simulink model "mod3_thermalnoises"  (R2013a)
settings: Solver=FixedStepDiscrete  StartTime=0.0  StopTime=swpctrl.trantime  RelTol=1e-3
undefined symbols (not defined in the file): Fs, modctrl
libraries: dspsrcs4 x4, dspsigops x3
settings Model: Creator=amyles  LastModifiedBy=amyles
settings DataIOCC: LimitDataPoints=off  MaxDataPoints=50000  SignalLoggingSaveFormat=ModelDataLogs
settings OptimizationCC: InlineParams=on  ExpressionDepthLimit=2147483647
settings DebuggingCC: FcnCallInpInsideContextMsg=UseLocalSettings  StrictBusMsg=Warning
settings ModelReferenceCC: ModelReferenceNumInstancesAllowed=Single
settings GRTTargetCC: CombineOutputUpdateFcns=off  GRTInterface=on

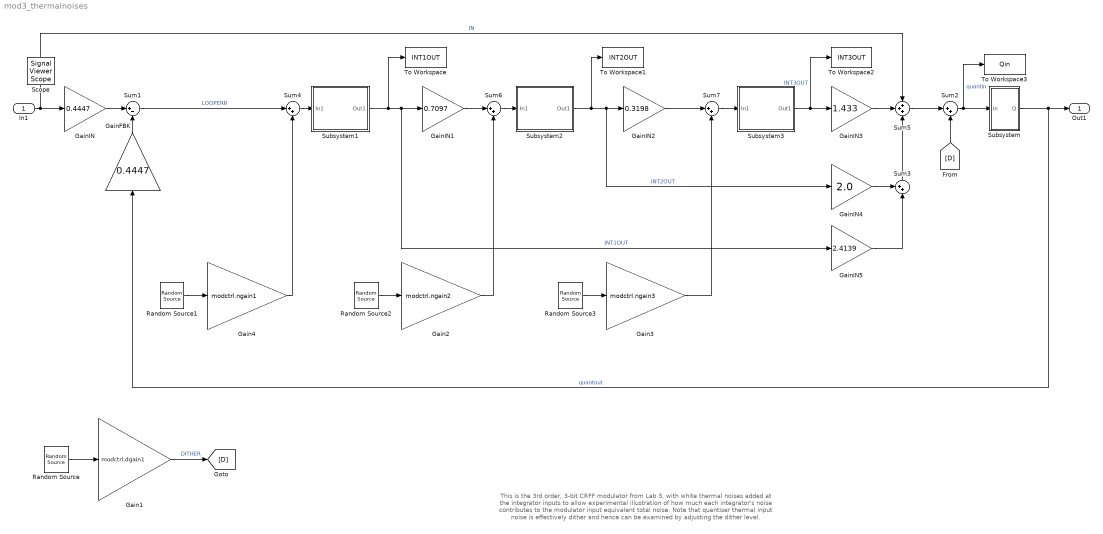
== system mod3_thermalnoises ==
  note: This is the 3rd order, 3-bit CRFF modulator from Lab 3, with
      | white thermal noises added at the integrator inputs to allow experimental
      | illustration of how much each integrator's noise contributes to the
      | modulator input equivalent total noise. Note that quantiser thermal input noise
      | is effectively dither and hence can be examined by adjusting the dither level.
  In1 : Inport
  Gain1 : Gain  Gain=modctrl.dgain1
      settings: AttributesFormatString=Dither level adjust
  Gain2 : Gain  Gain=modctrl.ngain2
  Gain3 : Gain  Gain=modctrl.ngain3
  Gain4 : Gain  Gain=modctrl.ngain1
  GainFBK : Gain  Gain=0.4447
  GainIN : Gain  Gain=0.4447
  GainIN1 : Gain  Gain=0.7097
  GainIN2 : Gain  Gain=0.3198
  GainIN3 : Gain  Gain=1.433
  GainIN4 : Gain  Gain=2.0
  GainIN5 : Gain  Gain=2.4139
  Random Source{,1..3} (4 alike) : dspsrcs4/Random Source  SrcType=Uniform  NormMethod=Ziggurat  CltLength=12  MinVal=-1  MaxVal=1  MeanVal=0  VarVal=1  RepMode=Not repeatable  rawSeed=1  IsInherit=off  SampMode=Discrete  SampTime=1/Fs  SampFrame=1  DataType=Double  OutComplex=Real
      Random Source settings: AttributesFormatString=Dither source
      Random Source1 settings: AttributesFormatString=INT1 noise
      Random Source2 settings: AttributesFormatString=INT1 noise
      Random Source3 settings: AttributesFormatString=INT1 noise
  Subsystem : Subsystem
      settings: AttributesFormatString=3-bit quantiser
  Subsystem1 : Subsystem
      settings: AttributesFormatString=Leaky delaying integrator
  Subsystem2 : Subsystem
      settings: AttributesFormatString=Leaky delayless integrator
  Subsystem3 : Subsystem
      settings: AttributesFormatString=Leaky delaying integrator
  Sum1 : Sum  Inputs=|+-
      settings: AttributesFormatString=Modulator input\nloop servo error (input - fbk)
  Sum{2,4,6..7} (4 alike) : Sum  Inputs=|++
  Sum3 : Sum  Inputs=++|
  Sum5 : Sum  Inputs=+++
  To Workspace : ToWorkspace  VariableName=INT1OUT  SampleTime=-1
  To Workspace1 : ToWorkspace  VariableName=INT2OUT  SampleTime=-1
  To Workspace2 : ToWorkspace  VariableName=INT3OUT  SampleTime=-1
  To Workspace3 : ToWorkspace  VariableName=Qin  SampleTime=-1
  Out1 : Outport
  Scope : SignalViewerScope  IOType=viewer  NumInputPorts=4  ZoomMode=xonly  RefreshTime=0.035000
      settings: YMin=-5~-5~-5~-5  YMax=5~5~5~5
  wires:
  Sum1/1 -> Sum4/1  "LOOPERR"
  In1/1 -> GainIN/1, Sum5/1  "IN"
  Sum2/1 -> Subsystem/1(in), To Workspace3/1  "quantin"
  Subsystem/1(Q) -> Out1/1, GainFBK/1  "quantout"
  Random Source/1 -> Gain1/1
  Subsystem1/1(Out1) -> GainIN1/1, GainIN5/1, To Workspace/1  "INT1OUT"
  GainIN1/1 -> Sum6/1
  Subsystem2/1(Out1) -> GainIN2/1, GainIN4/1, To Workspace1/1  "INT2OUT"
  Gain1/1 -> [D]  "DITHER"
  GainFBK/1 -> Sum1/2
  GainIN/1 -> Sum1/1
  Subsystem3/1(Out1) -> GainIN3/1, To Workspace2/1  "INT3OUT"
  Sum5/1 -> Sum2/1
  [D] -> Sum2/2
  GainIN2/1 -> Sum7/1
  GainIN3/1 -> Sum5/2
  GainIN4/1 -> Sum3/1
  Sum3/1 -> Sum5/3
  GainIN5/1 -> Sum3/2
  Random Source1/1 -> Gain4/1
  Gain4/1 -> Sum4/2
  Sum4/1 -> Subsystem1/1(In1)
  Sum6/1 -> Subsystem2/1(In1)
  Random Source2/1 -> Gain2/1
  Gain2/1 -> Sum6/2
  Sum7/1 -> Subsystem3/1(In1)
  Random Source3/1 -> Gain3/1
  Gain3/1 -> Sum7/2

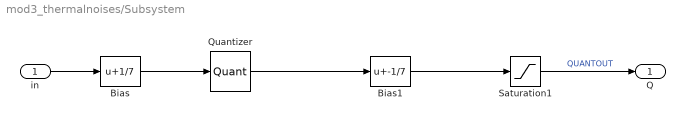
== system mod3_thermalnoises/Subsystem ==
  in : Inport
  Bias : Bias  Bias=1/7
      settings: AttributesFormatString=Need offset to give\nMID-RISE quantiser
  Bias1 : Bias  Bias=-1/7
  Quantizer : Quantizer  QuantizationInterval=2/7  LinearizeAsGain=off
  Saturation1 : Saturate  UpperLimit=1  LowerLimit=-1
      settings: AttributesFormatString=Limit quantiser\noutput to +/-1
  Q : Outport
  wires:
  Bias/1 -> Quantizer/1
  Quantizer/1 -> Bias1/1
  Bias1/1 -> Saturation1/1
  in/1 -> Bias/1
  Saturation1/1 -> Q/1  "QUANTOUT"

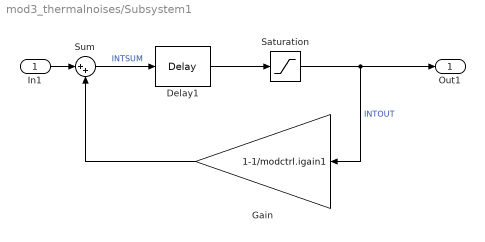
== system mod3_thermalnoises/Subsystem1 ==
  In1 : Inport
  Delay1 : dspsigops/Delay  dly_unit=Samples  delay=1  ic_detail=off  dif_ic_for_ch=off  dif_ic_for_dly=off  ic=0  reset_popup=None
  Gain : Gain  Gain=1-1/modctrl.igain1
      settings: AttributesFormatString=Integrator leakage
  Saturation : Saturate  UpperLimit=modctrl.isat1  LowerLimit=-(modctrl.isat1)
  Sum : Sum  Inputs=|++
      settings: AttributesFormatString=Integrator summer
  Out1 : Outport
  wires:
  Sum/1 -> Delay1/1  "INTSUM"
  Gain/1 -> Sum/2
  Saturation/1 -> Gain/1, Out1/1  "INTOUT"
  In1/1 -> Sum/1
  Delay1/1 -> Saturation/1

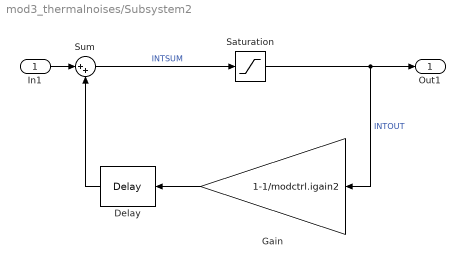
== system mod3_thermalnoises/Subsystem2 ==
  In1 : Inport
  Delay : dspsigops/Delay  dly_unit=Samples  delay=1  ic_detail=off  dif_ic_for_ch=off  dif_ic_for_dly=off  ic=0  reset_popup=None
  Gain : Gain  Gain=1-1/modctrl.igain2
      settings: AttributesFormatString=Integrator leakage
  Saturation : Saturate  UpperLimit=modctrl.isat2  LowerLimit=-(modctrl.isat2)
  Sum : Sum  Inputs=|++
      settings: AttributesFormatString=Integrator summer
  Out1 : Outport
  wires:
  In1/1 -> Sum/1
  Saturation/1 -> Out1/1, Gain/1  "INTOUT"
  Gain/1 -> Delay/1
  Sum/1 -> Saturation/1  "INTSUM"
  Delay/1 -> Sum/2

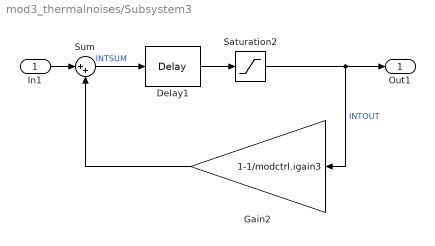
== system mod3_thermalnoises/Subsystem3 ==
  In1 : Inport
  Delay1 : dspsigops/Delay  dly_unit=Samples  delay=1  ic_detail=off  dif_ic_for_ch=off  dif_ic_for_dly=off  ic=0  reset_popup=None
  Gain2 : Gain  Gain=1-1/modctrl.igain3
      settings: AttributesFormatString=Integrator leakage
  Saturation2 : Saturate  UpperLimit=modctrl.isat3  LowerLimit=-(modctrl.isat3)
  Sum : Sum  Inputs=|++
      settings: AttributesFormatString=Integrator summer
  Out1 : Outport
  wires:
  Sum/1 -> Delay1/1  "INTSUM"
  Gain2/1 -> Sum/2
  Saturation2/1 -> Gain2/1, Out1/1  "INTOUT"
  In1/1 -> Sum/1
  Delay1/1 -> Saturation2/1
